simulink model "p1_MCU"  (R2023a)
settings: Solver=FixedStepDiscrete  StartTime=0.0  StopTime=inf  FixedStep=Ts_MCU  RelTol=1e-3  EnableMultiTasking=on
PreLoadFcn:
  | p1_params_new
  | spiDataDefinition
InitFcn:
  | mbd_s32k_consistency_checks(bdroot(gcs));
undefined symbols (not defined in the file or in its folder): ack, cpr_handwheel, cpr_steering, Discrete, DriverInput, DrivetrainLeft, DrivetrainRight, LQFP, MPU_IO, n_handwheel, n_steering, p1data, p1params, param, sr, steering_limit, SteeringLeft, SteeringRight, Time, Ts_MCU, wc, WheelForceLeft, WheelForceRight
libraries: simulink x74, mbd_s32k1xx_ec_toolbox x58, Library_Drivetrain x5, Library_Steering x5, etargetslib x3, ctrlSharedLib x1
(part 4 of 4)

== system p1_MCU/Steering Control/Steering Controller/HAL-9000/Latch ==
  In1 : Inport
  Trigger : TriggerPort  VariantControl=(inherit)
  Out1 : Outport
  wires:
  In1/1 -> Out1/1

== system p1_MCU/Steering Control/Steering Controller/HAL-9000/Ramp ==
  Start Time : Inport
  Digital Clock : DigitalClock  SampleTime=Ts_MCU
  Saturation : Saturate  UpperLimit=1  LowerLimit=0
  Slope : Gain  Gain=1/duration
  Sum : Sum  DisableCoverage=on  Inputs=|+-  InputSameDT=on  SaturateOnIntegerOverflow=on  OutDataTypeStr=Inherit: Same as first input
  Out1 : Outport
  wires:
  Slope/1 -> Saturation/1
  Saturation/1 -> Out1/1
  Sum/1 -> Slope/1
  Start Time/1 -> Sum/2
  Digital Clock/1 -> Sum/1

== system p1_MCU/Steering Control/Steering Controller/HAL-9000/Step ==
  Start Time : Inport
  Digital Clock : DigitalClock  SampleTime=Ts_MCU
  Relational Operator : RelationalOperator  OutDataTypeStr=float('double')  InputSameDT=off
  Out : Outport
  wires:
  Start Time/1 -> Relational Operator/2
  Digital Clock/1 -> Relational Operator/1
  Relational Operator/1 -> Out/1

== system p1_MCU/Steering Control/Steering Controller/HAL-9000/Double chirp/Chirp One ==
  note: freqSlope = deltaFreq/targetTime;
      | instantaneousFreq(t) = freqSlope*t + initialFreq;
      | intantaneousPhase(t) = integral(instFreq) = ...
      |       0.5*freqSlope*t^2 + initialFreq*t;
      | outputSignal(t) = sin(instantaneousPhase(t));
  Start Time : Inport
  Digital Clock : DigitalClock  SampleTime=Ts_MCU
  Gain : Gain  DisableCoverage=on  Gain=0.5  OutDataTypeStr=Inherit: Same as input  ParamDataTypeStr=Inherit: Same as input
  Output : Trigonometry
  Product : Product  DisableCoverage=on  Inputs=*/  InputSameDT=on  SaturateOnIntegerOverflow=on  OutDataTypeStr=Inherit: Same as first input
  Product1 : Product  DisableCoverage=on  InputSameDT=on  SaturateOnIntegerOverflow=on  OutDataTypeStr=Inherit: Same as first input
  Product2 : Product  DisableCoverage=on  InputSameDT=on  SaturateOnIntegerOverflow=on  OutDataTypeStr=Inherit: Same as first input
  Saturation : Saturate  UpperLimit=duration/2  LowerLimit=0
  Sum : Sum  DisableCoverage=on  Inputs=|++  InputSameDT=on  SaturateOnIntegerOverflow=on  OutDataTypeStr=Inherit: Same as first input
  Sum1 : Sum  DisableCoverage=on  Inputs=-+|  InputSameDT=on  SaturateOnIntegerOverflow=on  OutDataTypeStr=Inherit: Same as first input
  deltaFreq : Constant  DisableCoverage=on  Value=2*pi*(f2-f1)
  initialFreq : Constant  DisableCoverage=on  Value=2*pi*f1
  targetTime : Constant  DisableCoverage=on  Value=T
  Out2 : Outport
  wires:
  Sum1/1 -> Saturation/1
  Digital Clock/1 -> Sum1/2
  Start Time/1 -> Sum1/1
  deltaFreq/1 -> Product/1
  targetTime/1 -> Product/2
  Product/1 -> Gain/1
  Gain/1 -> Product1/2
  Product1/1 -> Sum/1
  initialFreq/1 -> Sum/2
  Sum/1 -> Product2/2
  Product2/1 -> Output/1
  Output/1 -> Out2/1
  Saturation/1 -> Product1/1, Product2/1

== system p1_MCU/Steering Control/Steering Controller/HAL-9000/Double chirp/Chirp Two ==
  note: freqSlope = deltaFreq/targetTime;
      | instantaneousFreq(t) = freqSlope*t + initialFreq;
      | intantaneousPhase(t) = integral(instFreq) = ...
      |       0.5*freqSlope*t^2 + initialFreq*t;
      | outputSignal(t) = sin(instantaneousPhase(t));
  Start Time : Inport
  Digital Clock : DigitalClock  SampleTime=Ts_MCU
  Gain : Gain  DisableCoverage=on  Gain=0.5  OutDataTypeStr=Inherit: Same as input  ParamDataTypeStr=Inherit: Same as input
  Output : Trigonometry
  Product : Product  DisableCoverage=on  Inputs=*/  InputSameDT=on  SaturateOnIntegerOverflow=on  OutDataTypeStr=Inherit: Same as first input
  Product1 : Product  DisableCoverage=on  InputSameDT=on  SaturateOnIntegerOverflow=on  OutDataTypeStr=Inherit: Same as first input
  Product2 : Product  DisableCoverage=on  InputSameDT=on  SaturateOnIntegerOverflow=on  OutDataTypeStr=Inherit: Same as first input
  Saturation : Saturate  UpperLimit=duration/2  LowerLimit=0
  Sum : Sum  DisableCoverage=on  Inputs=|++  InputSameDT=on  SaturateOnIntegerOverflow=on  OutDataTypeStr=Inherit: Same as first input
  Sum1 : Sum  DisableCoverage=on  Inputs=-+|  InputSameDT=on  SaturateOnIntegerOverflow=on  OutDataTypeStr=Inherit: Same as first input
  deltaFreq : Constant  DisableCoverage=on  Value=2*pi*(f2-f1)
  initialFreq : Constant  DisableCoverage=on  Value=2*pi*f1
  targetTime : Constant  DisableCoverage=on  Value=T
  Out2 : Outport
  wires:
  Sum1/1 -> Saturation/1
  Digital Clock/1 -> Sum1/2
  Start Time/1 -> Sum1/1
  deltaFreq/1 -> Product/1
  targetTime/1 -> Product/2
  Product/1 -> Gain/1
  Gain/1 -> Product1/2
  Product1/1 -> Sum/1
  initialFreq/1 -> Sum/2
  Sum/1 -> Product2/2
  Product2/1 -> Output/1
  Output/1 -> Out2/1
  Saturation/1 -> Product1/1, Product2/1
